simulink model "V7_Bearing_Vibration_Model"  (R2021b)
settings: Solver=ode3  StartTime=0  StopTime=1  FixedStep=1E-5  RelTol=1e-6
values from neighbouring files (symbols this model uses):
  D = 0.03932    [V8_tunedParameters.mat]
  d = 0.00794    [V8_tunedParameters.mat]
  excentricity = 4.24413e-06    [V8_tunedParameters.mat]
settings Model: Creator=PhilippSchildt  LastModifiedBy=PhilippSchildt
settings SolverCC: AlgebraicLoopSolver=TrustRegion
settings DebuggingCC: SFMachineParentedDataDiag=warning

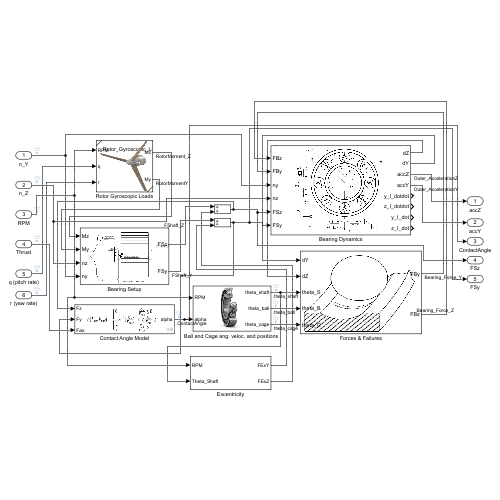
[thumbnail: Simulink's stored preview of the top-level diagram]
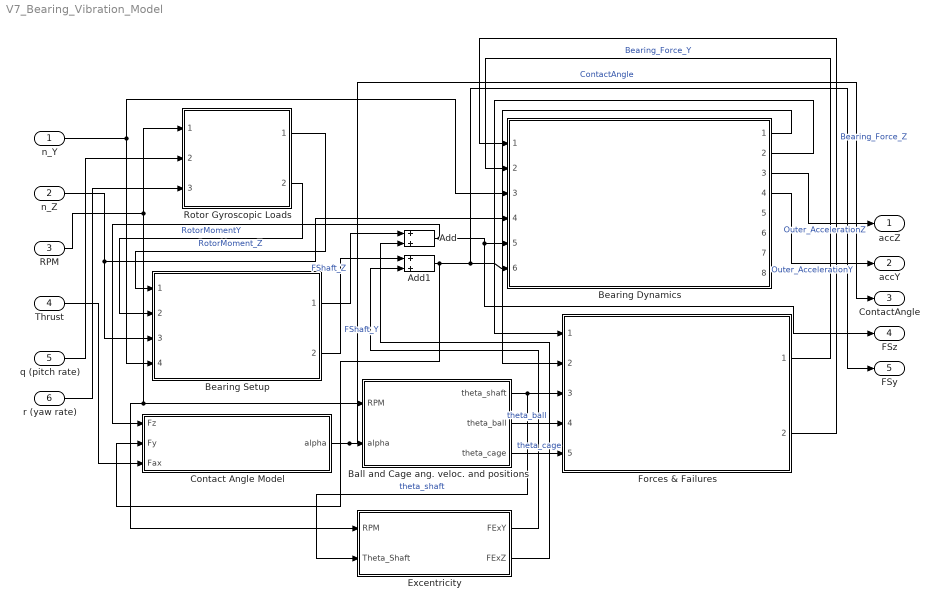
== system V7_Bearing_Vibration_Model ==
  n_Y : Inport
  n_Z : Inport  Port=2
  RPM : Inport  Port=3
  Thrust : Inport  Port=4
  q (pitch rate) : Inport  Port=5
  r (yaw rate) : Inport  Port=6
  Add : Sum
  Add1 : Sum
  "Ball and Cage ang. veloc. and positions " : Subsystem
      mask Display: image('$imagefile'); % Use "Edit Image" on toolstrip to change.
  Bearing Dynamics : Subsystem  ReferencedSubsystem=Bearing_Dynamics
  Bearing Setup : Subsystem  VariantControl=Choice  ReferencedSubsystem=Bearing_Setup
  Contact Angle Model : Subsystem
      mask Display: image('$imagefile'); % Use "Edit Image" on toolstrip to change.
  Excentricity : Subsystem
  Forces & Failures : Subsystem  ReferencedSubsystem=Bearing_Forces_Simulink_6307
  Rotor Gyroscopic Loads : Subsystem  ReferencedSubsystem=Rotor_Gyroscopic_Loads
  accZ : Outport
  accY : Outport  Port=2
  ContactAngle : Outport  Port=3
  FSz : Outport  Port=4
  FSy : Outport  Port=5
  wires:
  n_Z/1 -> Bearing Setup/3, Bearing Dynamics/4
  n_Y/1 -> Bearing Dynamics/3, Bearing Setup/4
  Contact Angle Model/1(alpha) -> ContactAngle/1, "Ball and Cage ang. veloc. and positions "/2(alpha)  "ContactAngle"
  Thrust/1 -> Contact Angle Model/3(Fax)
  RPM/1 -> "Ball and Cage ang. veloc. and positions "/1(RPM), Excentricity/1(RPM), Rotor Gyroscopic Loads/1
  "Ball and Cage ang. veloc. and positions "/3(theta_cage) -> Forces & Failures/5  "theta_cage"
  "Ball and Cage ang. veloc. and positions "/2(theta_ball) -> Forces & Failures/4  "theta_ball"
  "Ball and Cage ang. veloc. and positions "/1(theta_shaft) -> Excentricity/2(Theta_Shaft), Forces & Failures/3  "theta_shaft"
  Bearing Dynamics/3 -> accZ/1  "Outer_AccelerationZ"
  Bearing Dynamics/4 -> accY/1  "Outer_AccelerationY"
  Forces & Failures/1 -> Bearing Dynamics/2  "Bearing_Force_Y"
  Forces & Failures/2 -> Bearing Dynamics/1  "Bearing_Force_Z"
  Bearing Dynamics/1 -> Forces & Failures/2
  Bearing Dynamics/2 -> Forces & Failures/1
  Bearing Setup/1 -> Add/1  "FShaft_Z"
  Bearing Setup/2 -> Add1/1  "FShaft_Y"
  Add/1 -> Contact Angle Model/1(Fz), FSz/1, Bearing Dynamics/5
  Add1/1 -> Contact Angle Model/2(Fy), FSy/1, Bearing Dynamics/6
  Excentricity/1(FExY) -> Add1/2
  Excentricity/2(FExZ) -> Add/2
  q (pitch rate)/1 -> Rotor Gyroscopic Loads/2
  r (yaw rate)/1 -> Rotor Gyroscopic Loads/3
  Rotor Gyroscopic Loads/1 -> Bearing Setup/1  "RotorMoment_Z"
  Rotor Gyroscopic Loads/2 -> Bearing Setup/2  "RotorMomentY"

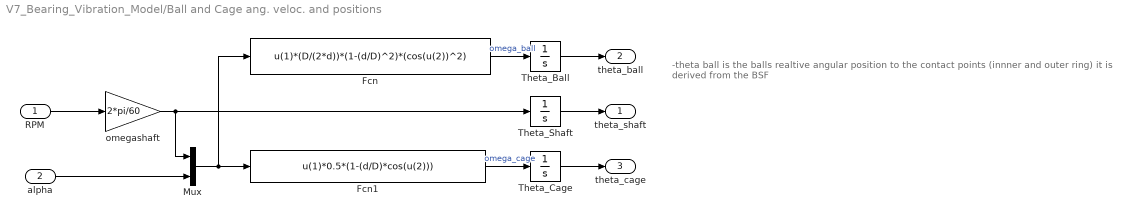
== system V7_Bearing_Vibration_Model/Ball and Cage ang. veloc. and positions  ==
  note: -theta ball is the balls realtive angular position to the contact points (innner and outer ring)
      | it is derived from the BSF
  RPM : Inport
  alpha : Inport  Port=2
  Fcn : Fcn  Expr=u(1)*(D/(2*d))*(1-(d/D)^2)*(cos(u(2))^2)
  Fcn1 : Fcn  Expr=u(1)*0.5*(1-(d/D)*cos(u(2)))
  Mux : Mux  Inputs=2
  Theta_Ball : Integrator  WrapState=on  WrappedStateUpperValue=2*pi()  WrappedStateLowerValue=0
  Theta_Cage : Integrator  WrapState=on  WrappedStateUpperValue=2*pi()  WrappedStateLowerValue=0
  Theta_Shaft : Integrator  WrapState=on  WrappedStateUpperValue=2*pi()  WrappedStateLowerValue=0
  omegashaft : Gain  Gain=2*pi/60
  theta_shaft : Outport
  theta_ball : Outport  Port=2
  theta_cage : Outport  Port=3
  wires:
  RPM/1 -> omegashaft/1
  Theta_Ball/1 -> theta_ball/1
  Theta_Shaft/1 -> theta_shaft/1
  Theta_Cage/1 -> theta_cage/1
  omegashaft/1 -> Mux/1, Theta_Shaft/1
  alpha/1 -> Mux/2
  Fcn1/1 -> Theta_Cage/1  "omega_cage"
  Fcn/1 -> Theta_Ball/1  "omega_ball"
  Mux/1 -> Fcn/1, Fcn1/1

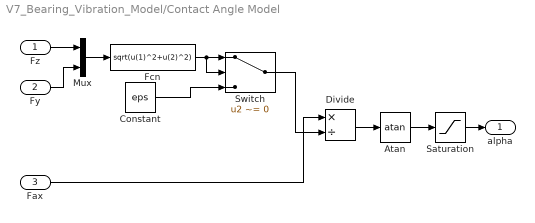
== system V7_Bearing_Vibration_Model/Contact Angle Model ==
  Fz : Inport
  Fy : Inport  Port=2
  Fax : Inport  Port=3
  Atan : Trigonometry  Operator=atan
  Constant : Constant  Value=eps
  Divide : Product  Inputs=*/
  Fcn : Fcn  Expr=sqrt(u(1)^2+u(2)^2)
  Mux : Mux  Inputs=2
  Saturation : Saturate  UpperLimit=pi/4  LowerLimit=0
  Switch : Switch  Criteria=u2 ~= 0
  alpha : Outport
  wires:
  Fz/1 -> Mux/1
  Constant/1 -> Switch/3
  Switch/1 -> Divide/2
  Fax/1 -> Divide/1
  Divide/1 -> Atan/1
  Atan/1 -> Saturation/1
  Saturation/1 -> alpha/1
  Fy/1 -> Mux/2
  Mux/1 -> Fcn/1
  Fcn/1 -> Switch/1, Switch/2

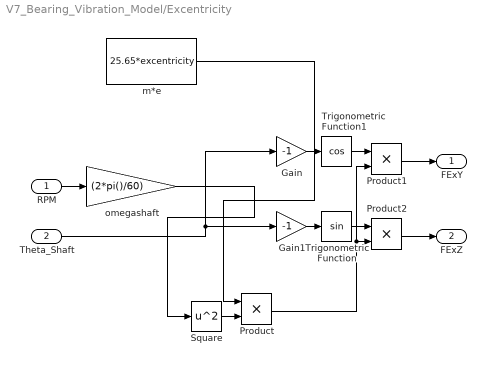
== system V7_Bearing_Vibration_Model/Excentricity ==
  RPM : Inport
  Theta_Shaft : Inport  Port=2
  Gain : Gain  Gain=-1
  Gain1 : Gain  Gain=-1
  Product : Product
  Product1 : Product
  Product2 : Product
  Square : Math  Operator=square  SaturateOnIntegerOverflow=on
  Trigonometric Function : Trigonometry
  Trigonometric Function1 : Trigonometry  Operator=cos
  m*e : Constant  Value=25.65*excentricity
  omegashaft : Gain  Gain=(2*pi()/60)
  FExY : Outport
  FExZ : Outport  Port=2
  wires:
  RPM/1 -> omegashaft/1
  m*e/1 -> Product/1
  Product2/1 -> FExZ/1
  Product1/1 -> FExY/1
  Trigonometric Function1/1 -> Product1/1
  Product/1 -> Product1/2, Product2/2
  Gain/1 -> Trigonometric Function1/1
  Theta_Shaft/1 -> Gain1/1, Gain/1
  Gain1/1 -> Trigonometric Function/1
  Trigonometric Function/1 -> Product2/1
  omegashaft/1 -> Square/1
  Square/1 -> Product/2
